simulink model "Subsystem"  (R2019b)
settings: Solver=FixedStepAuto  StartTime=0.0  StopTime=testtime  RelTol=1e-3
InitFcn:
  | Middle_Ear_Test_Parameters
StopFcn:
  | Verify_Middle_Ear
undefined symbols (not defined in the file or in its folder): MEcoeffs, MEscale
settings Model: Creator=mblun  LastModifiedBy=t96f346
settings DataIOCC: SaveOutput=off  SaveTime=off
settings OptimizationCC: BlockReduction=off  ConditionallyExecuteInputs=off  DefaultParameterBehavior=Inlined
settings DebuggingCC: AlgebraicLoopMsg=error
settings HardwareCC: ProdBitPerPointer=32  ProdBitPerSizeT=32  ProdBitPerPtrDiffT=32  ProdLargestAtomicFloat=None  ProdIntDivRoundTo=Undefined  ProdEndianess=Unspecified  ProdWordSize=32  ProdHWDeviceType=ASIC/FPGA->ASIC/FPGA  TargetBitPerPointer=64  TargetBitPerSizeT=64  TargetBitPerPtrDiffT=64  TargetLongLongMode=on  TargetIntDivRoundTo=Zero  TargetEndianess=LittleEndian  TargetWordSize=64  TargetHWDeviceType=Custom Processor->MATLAB Host Computer  ProdEqTarget=off
settings SFSimCC: CustomCodeUndefinedFunction=UseInterfaceOnly

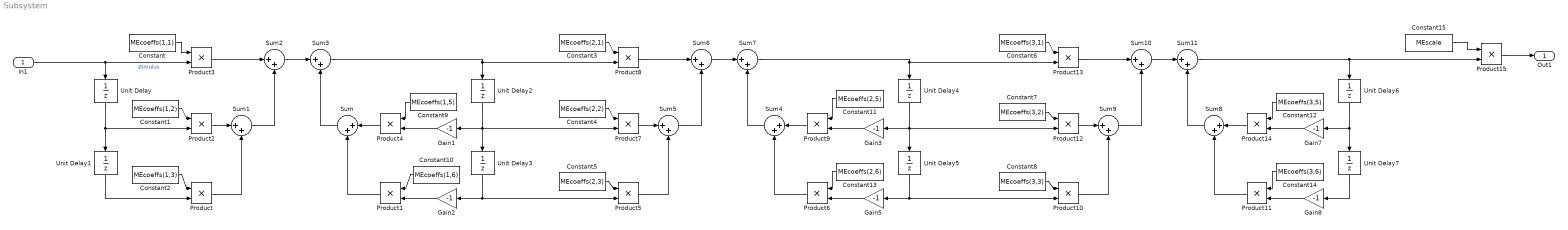
== system Subsystem ==
  In1 : Inport  OutDataTypeStr=single  PortDimensions=[1 1]  SampleTime=[2.0833333333333333e-05,0]
  Constant : Constant  Value=MEcoeffs(1,1)  OutDataTypeStr=single  SampleTime=-1
  Constant1 : Constant  Value=MEcoeffs(1,2)  OutDataTypeStr=single  SampleTime=-1
  Constant10 : Constant  Value=MEcoeffs(1,6)  OutDataTypeStr=single  SampleTime=-1
  Constant11 : Constant  Value=MEcoeffs(2,5)  OutDataTypeStr=single  SampleTime=-1
  Constant12 : Constant  Value=MEcoeffs(3,5)  OutDataTypeStr=single  SampleTime=-1
  Constant13 : Constant  Value=MEcoeffs(2,6)  OutDataTypeStr=single  SampleTime=-1
  Constant14 : Constant  Value=MEcoeffs(3,6)  OutDataTypeStr=single  SampleTime=-1
  Constant15 : Constant  Value=MEscale  OutDataTypeStr=single  SampleTime=-1
  Constant2 : Constant  Value=MEcoeffs(1,3)  OutDataTypeStr=single  SampleTime=-1
  Constant3 : Constant  Value=MEcoeffs(2,1)  OutDataTypeStr=single  SampleTime=-1
  Constant4 : Constant  Value=MEcoeffs(2,2)  OutDataTypeStr=single  SampleTime=-1
  Constant5 : Constant  Value=MEcoeffs(2,3)  OutDataTypeStr=single  SampleTime=-1
  Constant6 : Constant  Value=MEcoeffs(3,1)  OutDataTypeStr=single  SampleTime=-1
  Constant7 : Constant  Value=MEcoeffs(3,2)  OutDataTypeStr=single  SampleTime=-1
  Constant8 : Constant  Value=MEcoeffs(3,3)  OutDataTypeStr=single  SampleTime=-1
  Constant9 : Constant  Value=MEcoeffs(1,5)  OutDataTypeStr=single  SampleTime=-1
  Gain{1..3,5,7..8} (6 alike) : Gain  Gain=-1
  Product{,1..15} (16 alike) : Product
  Sum{,1..11} (12 alike) : Sum  Inputs=|++
  Unit Delay{,1..7} (8 alike) : UnitDelay  SampleTime=-1  HasFrameUpgradeWarning=on
  Out1 : Outport  OutDataTypeStr=single  PortDimensions=1  SampleTime=[2.0833333333333333e-05,0]
  wires:
  Product/1 -> Sum1/2
  Gain5/1 -> Product6/2
  Constant9/1 -> Product4/1
  Gain8/1 -> Product11/2
  Unit Delay1/1 -> Product/2
  Sum6/1 -> Sum7/1
  Gain2/1 -> Product1/2
  Product8/1 -> Sum6/1
  Gain3/1 -> Product9/2
  Sum10/1 -> Sum11/1
  Product9/1 -> Sum4/1
  Unit Delay6/1 -> Gain7/1, Unit Delay7/1
  Unit Delay3/1 -> Gain2/1, Product5/2
  Product6/1 -> Sum4/2
  Unit Delay5/1 -> Gain5/1, Product10/2
  Product13/1 -> Sum10/1
  Product5/1 -> Sum5/2
  Unit Delay7/1 -> Gain8/1
  Product2/1 -> Sum1/1
  Product14/1 -> Sum8/1
  Product10/1 -> Sum9/2
  Sum2/1 -> Sum3/1
  Sum11/1 -> Unit Delay6/1, Product15/2
  Unit Delay4/1 -> Gain3/1, Unit Delay5/1, Product12/2
  Product3/1 -> Sum2/1
  Sum/1 -> Sum3/2
  Sum3/1 -> Unit Delay2/1, Product8/2
  Product12/1 -> Sum9/1
  Sum8/1 -> Sum11/2
  Sum7/1 -> Unit Delay4/1, Product13/2
  Product7/1 -> Sum5/1
  Sum4/1 -> Sum7/2
  Sum5/1 -> Sum6/2
  In1/1 -> Unit Delay/1, Product3/2  "stimulus"
  Sum9/1 -> Sum10/2
  Unit Delay2/1 -> Gain1/1, Unit Delay3/1, Product7/2
  Constant/1 -> Product3/1
  Product1/1 -> Sum/2
  Sum1/1 -> Sum2/2
  Product11/1 -> Sum8/2
  Gain1/1 -> Product4/2
  Product4/1 -> Sum/1
  Gain7/1 -> Product14/2
  Unit Delay/1 -> Product2/2, Unit Delay1/1
  Constant1/1 -> Product2/1
  Constant3/1 -> Product8/1
  Constant4/1 -> Product7/1
  Constant5/1 -> Product5/1
  Constant6/1 -> Product13/1
  Constant7/1 -> Product12/1
  Constant8/1 -> Product10/1
  Constant2/1 -> Product/1
  Constant10/1 -> Product1/1
  Constant11/1 -> Product9/1
  Constant13/1 -> Product6/1
  Constant14/1 -> Product11/1
  Constant12/1 -> Product14/1
  Constant15/1 -> Product15/1
  Product15/1 -> Out1/1
